simulink model "Vehicle_long_dyn"  (R2020b)
settings: Solver=VariableStepAuto  StartTime=0.0  StopTime=300  RelTol=1e-3
values from neighbouring files (symbols this model uses):
  A = 2.24    [Vehicle_longitudinal_dynamics.m]
  Cd = 0.3    [Vehicle_longitudinal_dynamics.m]
  f = 0.0125    [Vehicle_longitudinal_dynamics.m]
  g = 9.81    [Vehicle_longitudinal_dynamics.m]
  m = 1084    [Vehicle_longitudinal_dynamics.m]
  rho = 1.2    [Vehicle_longitudinal_dynamics.m]
  Vw_0 = 1.2    [Vehicle_longitudinal_dynamics.m]
settings Model: Creator=ChOm1  LastModifiedBy=ChOm1

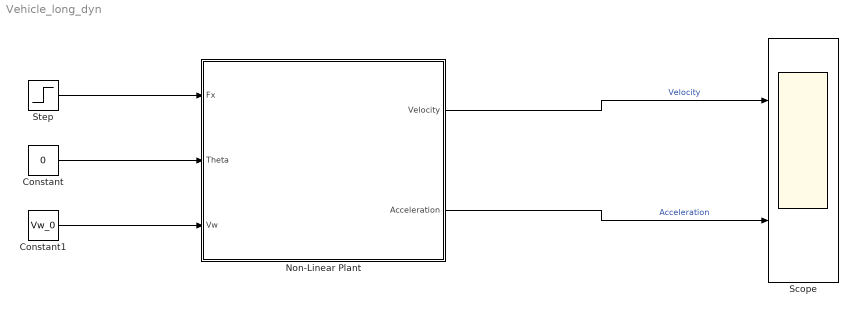
== system Vehicle_long_dyn ==
  Constant : Constant  Value=0
  Constant1 : Constant  Value=Vw_0
  Non-Linear Plant : Subsystem
  Scope : Scope  NumInputPorts=2
  Step : Step  SampleTime=0
  wires:
  Non-Linear Plant/1(Velocity) -> Scope/1  "Velocity"
  Non-Linear Plant/2(Acceleration) -> Scope/2  "Acceleration"
  Step/1 -> Non-Linear Plant/1(Fx)
  Constant/1 -> Non-Linear Plant/2(Theta)
  Constant1/1 -> Non-Linear Plant/3(Vw)

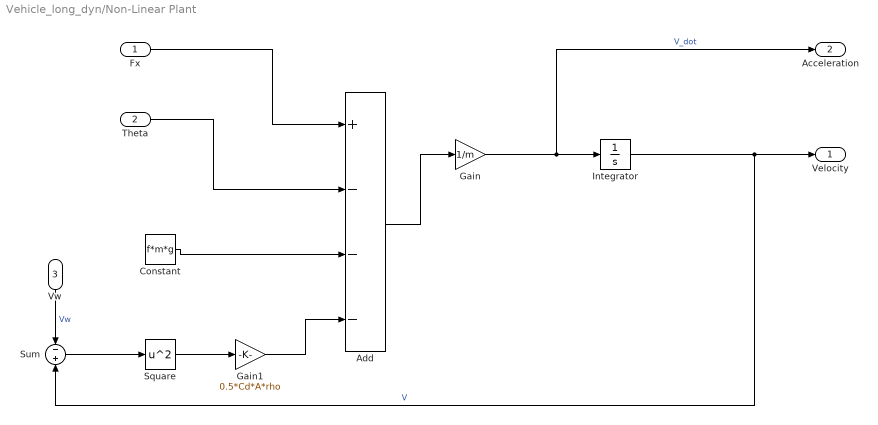
== system Vehicle_long_dyn/Non-Linear Plant ==
  Fx : Inport
  Theta : Inport  Port=2
  Vw : Inport  Port=3
  Add : Sum  Inputs=+---
  Constant : Constant  Value=f*m*g
  Gain : Gain  Gain=1/m
  Gain1 : Gain  Gain=0.5*Cd*A*rho
  Integrator : Integrator  InitialCondition=27.8
  Square : Math  Operator=square  SaturateOnIntegerOverflow=on
  Sum : Sum  Inputs=-+
  Velocity : Outport
  Acceleration : Outport  Port=2
  wires:
  Fx/1 -> Add/1
  Constant/1 -> Add/3
  Theta/1 -> Add/2
  Add/1 -> Gain/1
  Gain/1 -> Acceleration/1, Integrator/1  "V_dot"
  Integrator/1 -> Sum/2, Velocity/1  "V"
  Vw/1 -> Sum/1  "Vw"
  Sum/1 -> Square/1
  Square/1 -> Gain1/1
  Gain1/1 -> Add/4
